simulink model "boris"  (R2020b)
settings: Solver=ode5  StartTime=0.0  StopTime=inf  FixedStep=1.0  RelTol=1e-3  EnableMultiTasking=on
libraries: simulink_extras x8
settings Model: Creator=Administrator  LastModifiedBy=boris
settings DataIOCC: LimitDataPoints=on  SaveFormat=Array  SignalLoggingSaveFormat=ModelDataLogs  ReturnWorkspaceOutputs=off
settings OptimizationCC: InitFltsAndDblsToZero=on  LifeSpan=inf
settings DebuggingCC: SaveWithParameterizedLinksMsg=none  UnderspecifiedInitializationDetection=Classic  MergeDetectMultiDrivingBlocksExec=none  SignalResolutionControl=TryResolveAllWithWarning  SolverPrmCheckMsg=warning  FcnCallInpInsideContextMsg=warning  SFUnexpectedBacktrackingDiag=warning  SFNoUnconditionalDefaultTransitionDiag=warning  SFExecutionAtInitializationDiag=none  ArithmeticOperatorsInVariantConditions=warning
settings HardwareCC: ProdBitPerPointer=32  ProdBitPerSizeT=32  ProdBitPerPtrDiffT=32  ProdLargestAtomicFloat=None  ProdIntDivRoundTo=Undefined  ProdEndianess=Unspecified  ProdWordSize=32  ProdHWDeviceType=32-bit Generic  TargetHWDeviceType=32-bit Generic
settings ModelReferenceCC: PropagateSignalLabelsOutOfModel=off
settings SFSimCC: SimUseLocalCustomCode=off  CustomCodeUndefinedFunction=UseInterfaceOnly
settings RTWCC: RTWUseLocalCustomCode=off
settings CodeAppCC: StateflowObjectComments=on
settings GRTTargetCC: TargetFcnLib=ansi_tfl_tmw.mat  TargetLangStandard=C89/C90 (ANSI)  CombineOutputUpdateFcns=off  GRTInterface=on
settings ConfigComp: CovMetricSettings=dw  CovSaveCumulativeToWorkspaceVar=on  CovSaveSingleToWorkspaceVar=on  CovExternalEMLEnable=off

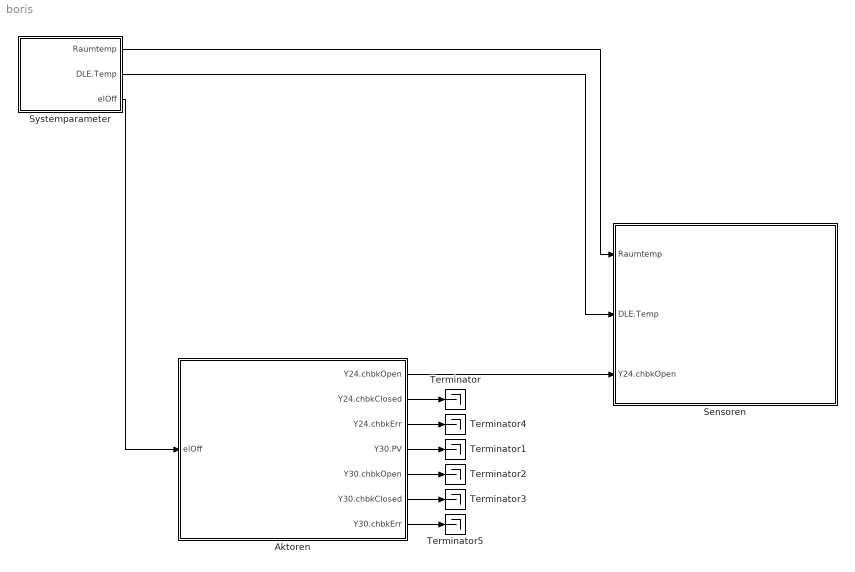
== system boris ==
  Aktoren : Subsystem  TreatAsAtomicUnit=on
  Sensoren : Subsystem  TreatAsAtomicUnit=on
  Systemparameter : Subsystem  TreatAsAtomicUnit=on
  Terminator{,1..5} (6 alike) : Terminator
  wires:
  Systemparameter/3(elOff) -> Aktoren/1(elOff)
  Systemparameter/2(DLE.Temp) -> Sensoren/2(DLE.Temp)
  Systemparameter/1(Raumtemp) -> Sensoren/1(Raumtemp)
  Aktoren/1(Y24.chbkOpen) -> Sensoren/3(Y24.chbkOpen)
  Aktoren/2(Y24.chbkClosed) -> Terminator/1
  Aktoren/4(Y30.PV) -> Terminator1/1
  Aktoren/5(Y30.chbkOpen) -> Terminator2/1
  Aktoren/6(Y30.chbkClosed) -> Terminator3/1
  Aktoren/3(Y24.chbkErr) -> Terminator4/1
  Aktoren/7(Y30.chbkErr) -> Terminator5/1

== system boris/Aktoren ==
  elOff : Inport  OutDataTypeStr=boolean
  Pumpen : Subsystem  TreatAsAtomicUnit=on
  Ventile : Subsystem  TreatAsAtomicUnit=on
  Y24.chbkOpen : Outport  OutDataTypeStr=boolean
  Y24.chbkClosed : Outport  Port=2  OutDataTypeStr=boolean
  Y24.chbkErr : Outport  Port=3  OutDataTypeStr=boolean
  Y30.PV : Outport  Port=4  OutDataTypeStr=double
  Y30.chbkOpen : Outport  Port=5  OutDataTypeStr=boolean
  Y30.chbkClosed : Outport  Port=6  OutDataTypeStr=boolean
  Y30.chbkErr : Outport  Port=7  OutDataTypeStr=boolean
  wires:
  elOff/1 -> Ventile/1(elOff), Pumpen/1(elOff)
  Ventile/1(Y24.chbkOpen) -> Y24.chbkOpen/1
  Ventile/2(Y24.chbkClosed) -> Y24.chbkClosed/1
  Ventile/4(Y30.PV) -> Y30.PV/1
  Ventile/6(Y30.chbkClosed) -> Y30.chbkClosed/1
  Ventile/5(Y30.chbkOpen) -> Y30.chbkOpen/1
  Ventile/3(Y24.chbkErr) -> Y24.chbkErr/1
  Ventile/7(Y30.chbkErr) -> Y30.chbkErr/1

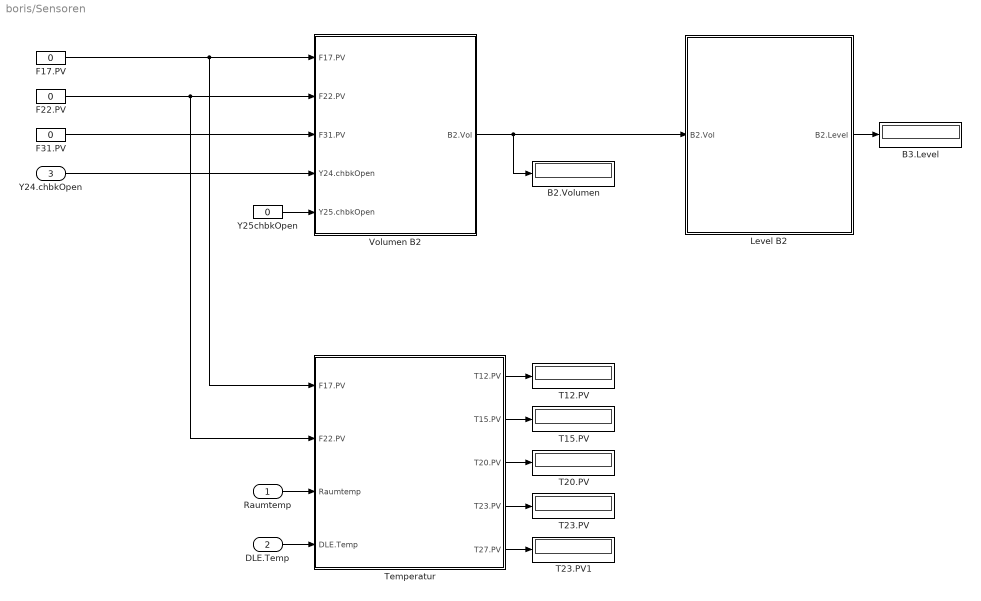
== system boris/Sensoren ==
  Raumtemp : Inport  OutDataTypeStr=double
  DLE.Temp : Inport  Port=2  OutDataTypeStr=double
  Y24.chbkOpen : Inport  Port=3  OutDataTypeStr=boolean
  B2.Volumen : Display
  B3.Level : Display
  F17.PV : Constant  Value=0  OutDataTypeStr=double
  F22.PV : Constant  Value=0  OutDataTypeStr=double
  F31.PV : Constant  Value=0  OutDataTypeStr=double
  Level B2 : Subsystem
  T12.PV : Display
  T15.PV : Display
  T20.PV : Display
  T23.PV : Display
  T23.PV1 : Display
  Temperatur : Subsystem
  Volumen B2 : Subsystem
  Y25chbkOpen : Constant  Value=0  OutDataTypeStr=boolean
  wires:
  Volumen B2/1(B2.Vol) -> Level B2/1(B2.Vol), B2.Volumen/1
  Raumtemp/1 -> Temperatur/3(Raumtemp)
  DLE.Temp/1 -> Temperatur/4(DLE.Temp)
  F17.PV/1 -> Volumen B2/1(F17.PV), Temperatur/1(F17.PV)
  F22.PV/1 -> Volumen B2/2(F22.PV), Temperatur/2(F22.PV)
  Y25chbkOpen/1 -> Volumen B2/5(Y25.chbkOpen)
  Temperatur/1(T12.PV) -> T12.PV/1
  Temperatur/2(T15.PV) -> T15.PV/1
  Temperatur/3(T20.PV) -> T20.PV/1
  Temperatur/4(T23.PV) -> T23.PV/1
  Level B2/1(B2.Level) -> B3.Level/1
  Y24.chbkOpen/1 -> Volumen B2/4(Y24.chbkOpen)
  F31.PV/1 -> Volumen B2/3(F31.PV)
  Temperatur/5(T27.PV) -> T23.PV1/1

== system boris/Systemparameter ==
  Ausfallwahrscheinlichkeit Stromversorgung : Constant  Value=0  OutDataTypeStr=double
  Ausgefallene Stromversorgung reparieren : Constant  Value=0  OutDataTypeStr=boolean
  Notaus : Constant  OutDataTypeStr=boolean
  Power : Constant  OutDataTypeStr=boolean
  Raumtemperatur : Constant  Value=20  OutDataTypeStr=double
  Strom aus? : Subsystem
  Temperatur Durchflauferhitzer : Constant  Value=40  OutDataTypeStr=double
  Raumtemp : Outport  OutDataTypeStr=double
  DLE.Temp : Outport  Port=2  OutDataTypeStr=double
  elOff : Outport  Port=3  OutDataTypeStr=boolean
  wires:
  Raumtemperatur/1 -> Raumtemp/1  "Raumtemp"
  Temperatur Durchflauferhitzer/1 -> DLE.Temp/1  "DLE.Temp"
  Notaus/1 -> Strom aus?/1(ilSSw)
  Power/1 -> Strom aus?/2(power)
  Ausfallwahrscheinlichkeit Stromversorgung/1 -> Strom aus?/3(pErrPow)
  Ausgefallene Stromversorgung reparieren/1 -> Strom aus?/4(PowRepai)
  Strom aus?/1(elOff) -> elOff/1  "elOff"

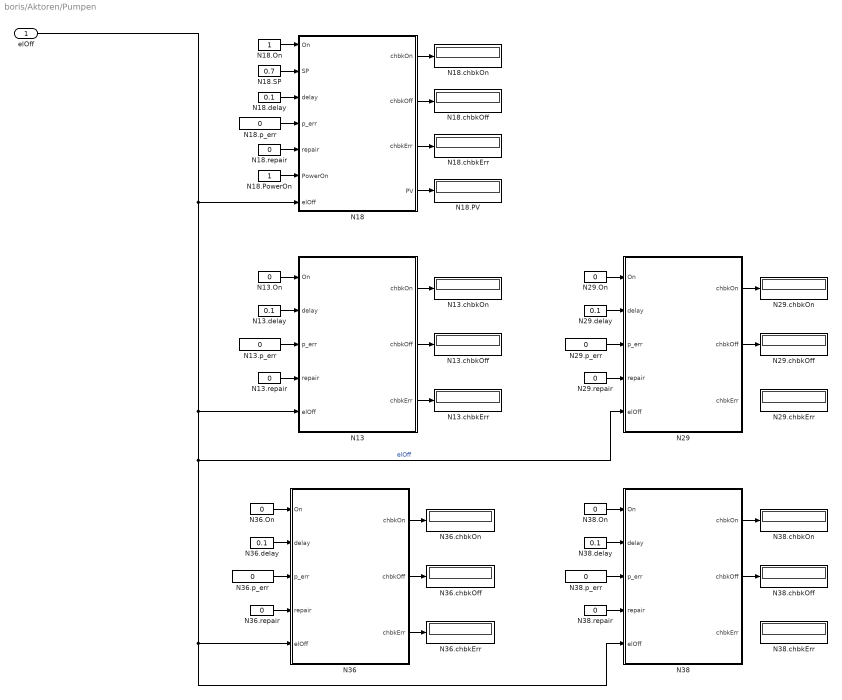
== system boris/Aktoren/Pumpen ==
  elOff : Inport  OutDataTypeStr=boolean
  N13 : Subsystem
  N13.On : Constant  Value=0  OutDataTypeStr=boolean
  N13.chbkErr : Display
  N13.chbkOff : Display
  N13.chbkOn : Display
  N13.delay : Constant  Value=0.1  OutDataTypeStr=double
  N13.p_err : Constant  Value=0  OutDataTypeStr=double
  N13.repair : Constant  Value=0  OutDataTypeStr=boolean
  N18 : Subsystem
  N18.On : Constant  OutDataTypeStr=boolean
  N18.PV : Display
  N18.PowerOn : Constant  OutDataTypeStr=boolean
  N18.SP : Constant  Value=0.7  OutDataTypeStr=double
  N18.chbkErr : Display
  N18.chbkOff : Display
  N18.chbkOn : Display
  N18.delay : Constant  Value=0.1  OutDataTypeStr=double
  N18.p_err : Constant  Value=0  OutDataTypeStr=double
  N18.repair : Constant  Value=0  OutDataTypeStr=boolean
  N29 : Subsystem
  N29.On : Constant  Value=0  OutDataTypeStr=boolean
  N29.chbkErr : Display
  N29.chbkOff : Display
  N29.chbkOn : Display
  N29.delay : Constant  Value=0.1  OutDataTypeStr=double
  N29.p_err : Constant  Value=0  OutDataTypeStr=double
  N29.repair : Constant  Value=0  OutDataTypeStr=boolean
  N36 : Subsystem
  N36.On : Constant  Value=0  OutDataTypeStr=boolean
  N36.chbkErr : Display
  N36.chbkOff : Display
  N36.chbkOn : Display
  N36.delay : Constant  Value=0.1  OutDataTypeStr=double
  N36.p_err : Constant  Value=0  OutDataTypeStr=double
  N36.repair : Constant  Value=0  OutDataTypeStr=boolean
  N38 : Subsystem
  N38.On : Constant  Value=0  OutDataTypeStr=boolean
  N38.chbkErr : Display
  N38.chbkOff : Display
  N38.chbkOn : Display
  N38.delay : Constant  Value=0.1  OutDataTypeStr=double
  N38.p_err : Constant  Value=0  OutDataTypeStr=double
  N38.repair : Constant  Value=0  OutDataTypeStr=boolean
  wires:
  N18/1(chbkOn) -> N18.chbkOn/1
  N18/2(chbkOff) -> N18.chbkOff/1
  N18/3(chbkErr) -> N18.chbkErr/1
  N18/4(PV) -> N18.PV/1
  N18.On/1 -> N18/1(On)
  N18.SP/1 -> N18/2(SP)
  N18.delay/1 -> N18/3(delay)
  N18.p_err/1 -> N18/4(p_err)
  N18.repair/1 -> N18/5(repair)
  N18.PowerOn/1 -> N18/6(PowerOn)
  N13/1(chbkOn) -> N13.chbkOn/1
  N13/2(chbkOff) -> N13.chbkOff/1
  N13.On/1 -> N13/1(On)
  N13.delay/1 -> N13/2(delay)
  N13.p_err/1 -> N13/3(p_err)
  N13.repair/1 -> N13/4(repair)
  N29/1(chbkOn) -> N29.chbkOn/1
  N29/2(chbkOff) -> N29.chbkOff/1
  ? -> N29.chbkErr/1
  N29.On/1 -> N29/1(On)
  N29.delay/1 -> N29/2(delay)
  N29.p_err/1 -> N29/3(p_err)
  N29.repair/1 -> N29/4(repair)
  N36/1(chbkOn) -> N36.chbkOn/1
  N36/2(chbkOff) -> N36.chbkOff/1
  N36/3(chbkErr) -> N36.chbkErr/1
  N36.On/1 -> N36/1(On)
  N36.delay/1 -> N36/2(delay)
  N36.p_err/1 -> N36/3(p_err)
  N36.repair/1 -> N36/4(repair)
  N38/1(chbkOn) -> N38.chbkOn/1
  N38/2(chbkOff) -> N38.chbkOff/1
  ? -> N38.chbkErr/1
  N38.On/1 -> N38/1(On)
  N38.delay/1 -> N38/2(delay)
  N38.p_err/1 -> N38/3(p_err)
  N38.repair/1 -> N38/4(repair)
  elOff/1 -> N13/5(elOff), N29/5(elOff), N36/5(elOff), N38/5(elOff), N18/7(elOff)  "elOff"
  N13/3(chbkErr) -> N13.chbkErr/1

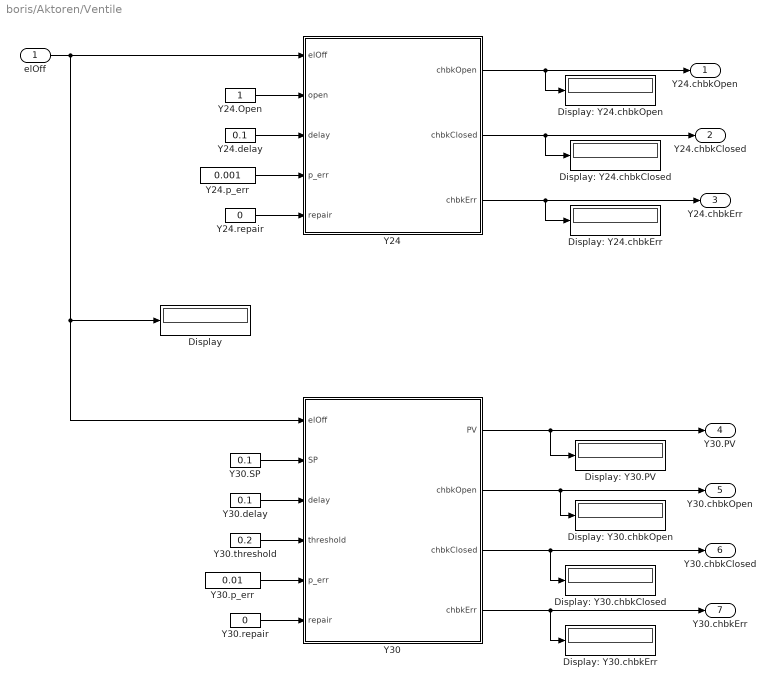
== system boris/Aktoren/Ventile ==
  elOff : Inport  OutDataTypeStr=boolean
  Display : Display
  Display: Y24.chbkClosed : Display
  Display: Y24.chbkErr : Display
  Display: Y24.chbkOpen : Display
  Display: Y30.PV : Display
  Display: Y30.chbkClosed : Display
  Display: Y30.chbkErr : Display
  Display: Y30.chbkOpen : Display
  Y24 : Subsystem
  Y24.Open : Constant  OutDataTypeStr=boolean
  Y24.delay : Constant  Value=0.1  OutDataTypeStr=double
  Y24.p_err : Constant  Value=0.001  OutDataTypeStr=double
  Y24.repair : Constant  Value=0  OutDataTypeStr=boolean
  Y30 : Subsystem
  Y30.SP : Constant  Value=0.1  OutDataTypeStr=double
  Y30.delay : Constant  Value=0.1  OutDataTypeStr=double
  Y30.p_err : Constant  Value=0.01  OutDataTypeStr=double
  Y30.repair : Constant  Value=0  OutDataTypeStr=boolean
  Y30.threshold : Constant  Value=0.2  OutDataTypeStr=double
  Y24.chbkOpen : Outport  OutDataTypeStr=boolean
  Y24.chbkClosed : Outport  Port=2  OutDataTypeStr=boolean
  Y24.chbkErr : Outport  Port=3  OutDataTypeStr=boolean
  Y30.PV : Outport  Port=4  OutDataTypeStr=double
  Y30.chbkOpen : Outport  Port=5  OutDataTypeStr=boolean
  Y30.chbkClosed : Outport  Port=6  OutDataTypeStr=boolean
  Y30.chbkErr : Outport  Port=7  OutDataTypeStr=boolean
  wires:
  elOff/1 -> Y24/1(elOff), Display/1, Y30/1(elOff)
  Y24.Open/1 -> Y24/2(open)
  Y24.delay/1 -> Y24/3(delay)
  Y24.p_err/1 -> Y24/4(p_err)
  Y24.repair/1 -> Y24/5(repair)
  Y30.SP/1 -> Y30/2(SP)
  Y30.delay/1 -> Y30/3(delay)
  Y30.p_err/1 -> Y30/5(p_err)
  Y30.repair/1 -> Y30/6(repair)
  Y30.threshold/1 -> Y30/4(threshold)
  Y24/1(chbkOpen) -> Display: Y24.chbkOpen/1, Y24.chbkOpen/1
  Y24/2(chbkClosed) -> Display: Y24.chbkClosed/1, Y24.chbkClosed/1
  Y30/1(PV) -> Display: Y30.PV/1, Y30.PV/1
  Y30/2(chbkOpen) -> Display: Y30.chbkOpen/1, Y30.chbkOpen/1
  Y30/3(chbkClosed) -> Display: Y30.chbkClosed/1, Y30.chbkClosed/1
  Y30/4(chbkErr) -> Display: Y30.chbkErr/1, Y30.chbkErr/1
  Y24/3(chbkErr) -> Display: Y24.chbkErr/1, Y24.chbkErr/1

== system boris/Sensoren/Level B2 ==
  B2.Vol : Inport
  B2.Level : Outport

== system boris/Sensoren/Temperatur ==
  F17.PV : Inport  OutDataTypeStr=double
  F22.PV : Inport  Port=2  OutDataTypeStr=double
  Raumtemp : Inport  Port=3  OutDataTypeStr=double
  DLE.Temp : Inport  Port=4  OutDataTypeStr=double
  T12.PV : Outport  OutDataTypeStr=double
  T15.PV : Outport  Port=2  OutDataTypeStr=double
  T20.PV : Outport  Port=3  OutDataTypeStr=double
  T23.PV : Outport  Port=4  OutDataTypeStr=double
  T27.PV : Outport  Port=5  OutDataTypeStr=double

== system boris/Sensoren/Volumen B2 ==
  F17.PV : Inport  OutDataTypeStr=double
  F22.PV : Inport  Port=2  OutDataTypeStr=double
  F31.PV : Inport  Port=3  OutDataTypeStr=double
  Y24.chbkOpen : Inport  Port=4  OutDataTypeStr=boolean
  Y25.chbkOpen : Inport  Port=5  OutDataTypeStr=boolean
  B2.Vol : Outport

== system boris/Systemparameter/Strom aus? ==
  ilSSw : Inport
  power : Inport  Port=2
  pErrPow : Inport  Port=3  OutDataTypeStr=double
  PowRepai : Inport  Port=4  OutDataTypeStr=boolean
  Logical Operator : Logic  AllPortsSameDT=off  OutDataTypeStr=boolean
  Logical Operator1 : Logic  Operator=NOT  AllPortsSameDT=off  OutDataTypeStr=boolean
  Notaus? : Subsystem  TreatAsAtomicUnit=on
  Stromausfall? : Subsystem  TreatAsAtomicUnit=on
  elOff : Outport  OutDataTypeStr=boolean
  wires:
  pErrPow/1 -> Stromausfall?/2(p_err)
  power/1 -> Stromausfall?/1(power), Notaus?/2(power)
  ilSSw/1 -> Notaus?/1(ilSSw)
  Logical Operator/1 -> Logical Operator1/1
  Notaus?/1(elOn) -> Logical Operator/1
  Stromausfall?/1(pow) -> Logical Operator/2
  PowRepai/1 -> Stromausfall?/3(repair)
  Logical Operator1/1 -> elOff/1

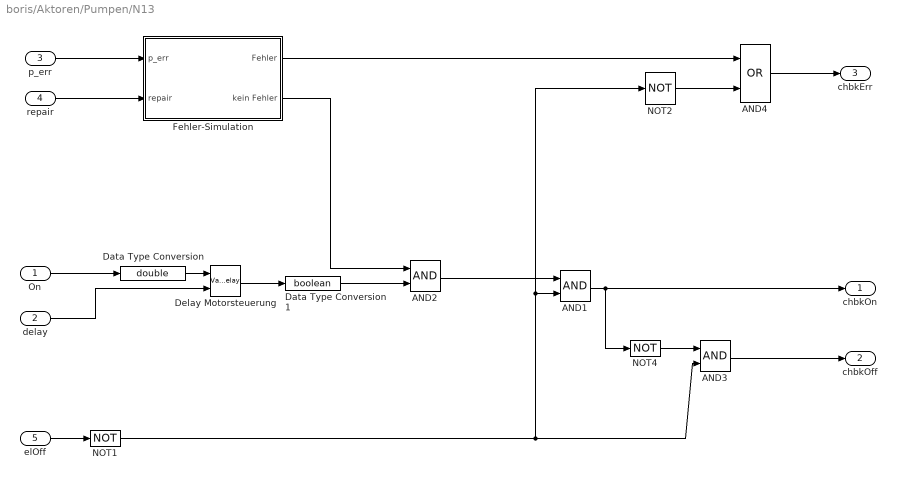
== system boris/Aktoren/Pumpen/N13 ==
  On : Inport  OutDataTypeStr=boolean
  delay : Inport  Port=2  OutDataTypeStr=double
  p_err : Inport  Port=3  OutDataTypeStr=double
  repair : Inport  Port=4  OutDataTypeStr=boolean
  elOff : Inport  Port=5  OutDataTypeStr=boolean
  AND1 : Logic  AllPortsSameDT=off  OutDataTypeStr=boolean
  AND2 : Logic  AllPortsSameDT=off  OutDataTypeStr=boolean
  AND3 : Logic  AllPortsSameDT=off  OutDataTypeStr=boolean
  AND4 : Logic  Operator=OR  AllPortsSameDT=off  OutDataTypeStr=boolean
  Data Type Conversion : DataTypeConversion  OutDataTypeStr=double
  Data Type Conversion1 : DataTypeConversion  OutDataTypeStr=boolean
  Delay Motorsteuerung : VariableTransportDelay  MaximumDelay=10  FixedBuffer=on
  Fehler-Simulation : Subsystem  TreatAsAtomicUnit=on
  NOT1 : Logic  Operator=NOT  AllPortsSameDT=off  OutDataTypeStr=boolean
  NOT2 : Logic  Operator=NOT  AllPortsSameDT=off  OutDataTypeStr=boolean
  NOT4 : Logic  Operator=NOT  AllPortsSameDT=off  OutDataTypeStr=boolean
  chbkOn : Outport  OutDataTypeStr=boolean
  chbkOff : Outport  Port=2  OutDataTypeStr=boolean
  chbkErr : Outport  Port=3  OutDataTypeStr=boolean
  wires:
  delay/1 -> Delay Motorsteuerung/2
  On/1 -> Data Type Conversion/1
  Delay Motorsteuerung/1 -> Data Type Conversion1/1
  Data Type Conversion/1 -> Delay Motorsteuerung/1
  Data Type Conversion1/1 -> AND2/2
  p_err/1 -> Fehler-Simulation/1(p_err)
  repair/1 -> Fehler-Simulation/2(repair)
  elOff/1 -> NOT1/1
  NOT1/1 -> AND3/2, AND1/2, NOT2/1
  AND2/1 -> AND1/1
  AND1/1 -> NOT4/1, chbkOn/1
  NOT4/1 -> AND3/1
  AND3/1 -> chbkOff/1
  Fehler-Simulation/2(kein Fehler) -> AND2/1
  AND4/1 -> chbkErr/1
  NOT2/1 -> AND4/2
  Fehler-Simulation/1(Fehler) -> AND4/1

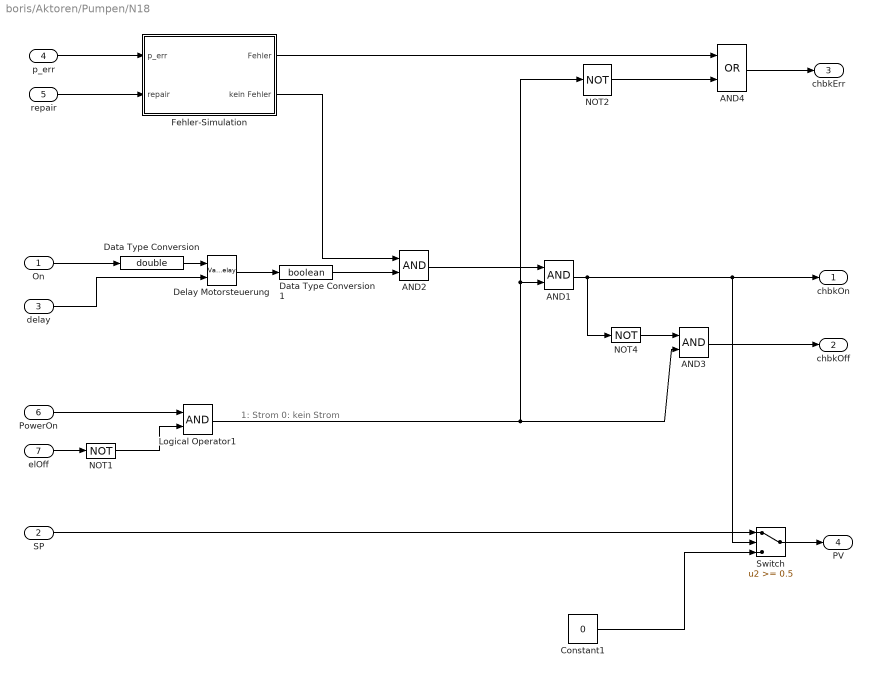
== system boris/Aktoren/Pumpen/N18 ==
  note: 1: Strom
      | 0: kein Strom
  On : Inport  OutDataTypeStr=boolean
  SP : Inport  Port=2  OutDataTypeStr=double
  delay : Inport  Port=3  OutDataTypeStr=double
  p_err : Inport  Port=4  OutDataTypeStr=double
  repair : Inport  Port=5  OutDataTypeStr=boolean
  PowerOn : Inport  Port=6  OutDataTypeStr=boolean
  elOff : Inport  Port=7  OutDataTypeStr=boolean
  AND1 : Logic  AllPortsSameDT=off  OutDataTypeStr=boolean
  AND2 : Logic  AllPortsSameDT=off  OutDataTypeStr=boolean
  AND3 : Logic  AllPortsSameDT=off  OutDataTypeStr=boolean
  AND4 : Logic  Operator=OR  AllPortsSameDT=off  OutDataTypeStr=boolean
  Constant1 : Constant  Value=0
  Data Type Conversion : DataTypeConversion  OutDataTypeStr=double
  Data Type Conversion1 : DataTypeConversion  OutDataTypeStr=boolean
  Delay Motorsteuerung : VariableTransportDelay  MaximumDelay=10  FixedBuffer=on
  Fehler-Simulation : Subsystem  TreatAsAtomicUnit=on
  Logical Operator1 : Logic  AllPortsSameDT=off  OutDataTypeStr=boolean
  NOT1 : Logic  Operator=NOT  AllPortsSameDT=off  OutDataTypeStr=boolean
  NOT2 : Logic  Operator=NOT  AllPortsSameDT=off  OutDataTypeStr=boolean
  NOT4 : Logic  Operator=NOT  AllPortsSameDT=off  OutDataTypeStr=boolean
  Switch : Switch  Threshold=0.5
  chbkOn : Outport  OutDataTypeStr=boolean
  chbkOff : Outport  Port=2  OutDataTypeStr=boolean
  chbkErr : Outport  Port=3  OutDataTypeStr=boolean
  PV : Outport  Port=4  OutDataTypeStr=double
  wires:
  delay/1 -> Delay Motorsteuerung/2
  On/1 -> Data Type Conversion/1
  Delay Motorsteuerung/1 -> Data Type Conversion1/1
  Logical Operator1/1 -> AND3/2, AND1/2, NOT2/1
  Data Type Conversion/1 -> Delay Motorsteuerung/1
  Data Type Conversion1/1 -> AND2/2
  p_err/1 -> Fehler-Simulation/1(p_err)
  repair/1 -> Fehler-Simulation/2(repair)
  PowerOn/1 -> Logical Operator1/1
  elOff/1 -> NOT1/1
  NOT1/1 -> Logical Operator1/2
  AND2/1 -> AND1/1
  AND1/1 -> NOT4/1, chbkOn/1, Switch/2
  NOT4/1 -> AND3/1
  AND3/1 -> chbkOff/1
  Fehler-Simulation/2(kein Fehler) -> AND2/1
  AND4/1 -> chbkErr/1
  Constant1/1 -> Switch/3
  Switch/1 -> PV/1
  SP/1 -> Switch/1
  NOT2/1 -> AND4/2
  Fehler-Simulation/1(Fehler) -> AND4/1

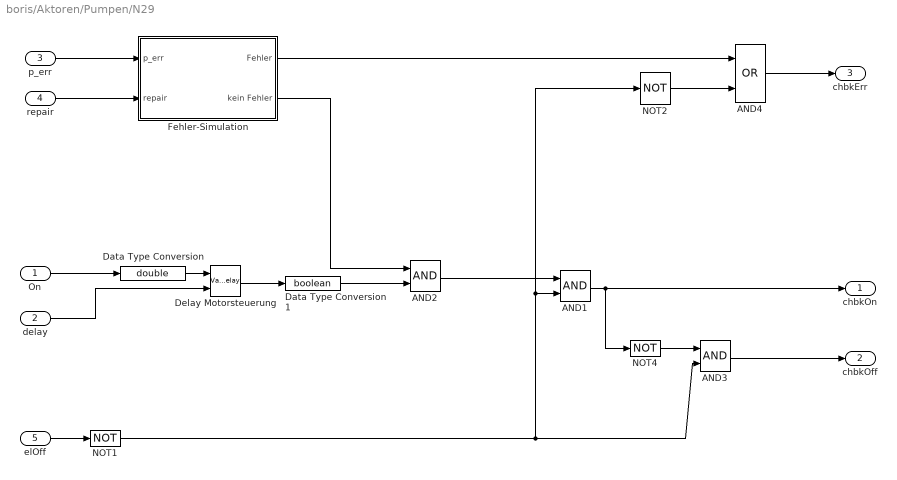
== system boris/Aktoren/Pumpen/N29 ==
  On : Inport  OutDataTypeStr=boolean
  delay : Inport  Port=2  OutDataTypeStr=double
  p_err : Inport  Port=3  OutDataTypeStr=double
  repair : Inport  Port=4  OutDataTypeStr=boolean
  elOff : Inport  Port=5  OutDataTypeStr=boolean
  AND1 : Logic  AllPortsSameDT=off  OutDataTypeStr=boolean
  AND2 : Logic  AllPortsSameDT=off  OutDataTypeStr=boolean
  AND3 : Logic  AllPortsSameDT=off  OutDataTypeStr=boolean
  AND4 : Logic  Operator=OR  AllPortsSameDT=off  OutDataTypeStr=boolean
  Data Type Conversion : DataTypeConversion  OutDataTypeStr=double
  Data Type Conversion1 : DataTypeConversion  OutDataTypeStr=boolean
  Delay Motorsteuerung : VariableTransportDelay  MaximumDelay=10  FixedBuffer=on
  Fehler-Simulation : Subsystem  TreatAsAtomicUnit=on
  NOT1 : Logic  Operator=NOT  AllPortsSameDT=off  OutDataTypeStr=boolean
  NOT2 : Logic  Operator=NOT  AllPortsSameDT=off  OutDataTypeStr=boolean
  NOT4 : Logic  Operator=NOT  AllPortsSameDT=off  OutDataTypeStr=boolean
  chbkOn : Outport  OutDataTypeStr=boolean
  chbkOff : Outport  Port=2  OutDataTypeStr=boolean
  chbkErr : Outport  Port=3  OutDataTypeStr=boolean
  wires:
  delay/1 -> Delay Motorsteuerung/2
  On/1 -> Data Type Conversion/1
  Delay Motorsteuerung/1 -> Data Type Conversion1/1
  Data Type Conversion/1 -> Delay Motorsteuerung/1
  Data Type Conversion1/1 -> AND2/2
  p_err/1 -> Fehler-Simulation/1(p_err)
  repair/1 -> Fehler-Simulation/2(repair)
  elOff/1 -> NOT1/1
  NOT1/1 -> AND3/2, AND1/2, NOT2/1
  AND2/1 -> AND1/1
  AND1/1 -> NOT4/1, chbkOn/1
  NOT4/1 -> AND3/1
  AND3/1 -> chbkOff/1
  Fehler-Simulation/2(kein Fehler) -> AND2/1
  AND4/1 -> chbkErr/1
  NOT2/1 -> AND4/2
  Fehler-Simulation/1(Fehler) -> AND4/1

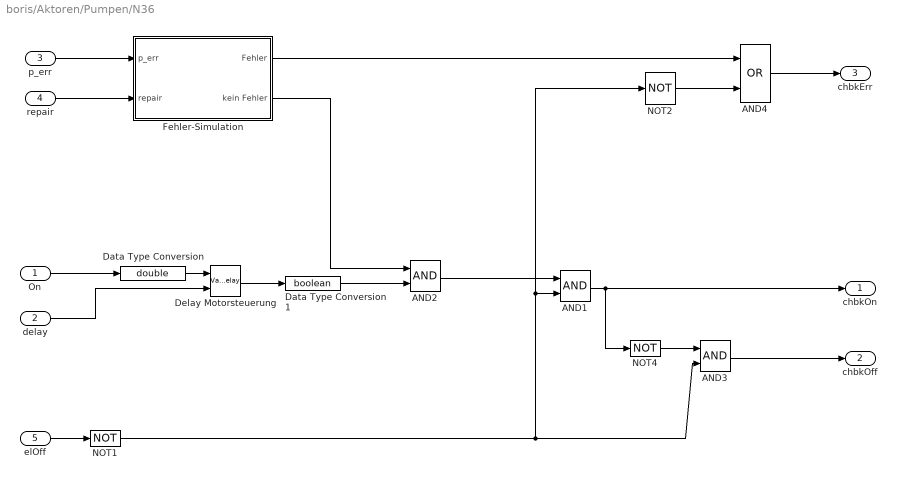
== system boris/Aktoren/Pumpen/N36 ==
  On : Inport  OutDataTypeStr=boolean
  delay : Inport  Port=2  OutDataTypeStr=double
  p_err : Inport  Port=3  OutDataTypeStr=double
  repair : Inport  Port=4  OutDataTypeStr=boolean
  elOff : Inport  Port=5  OutDataTypeStr=boolean
  AND1 : Logic  AllPortsSameDT=off  OutDataTypeStr=boolean
  AND2 : Logic  AllPortsSameDT=off  OutDataTypeStr=boolean
  AND3 : Logic  AllPortsSameDT=off  OutDataTypeStr=boolean
  AND4 : Logic  Operator=OR  AllPortsSameDT=off  OutDataTypeStr=boolean
  Data Type Conversion : DataTypeConversion  OutDataTypeStr=double
  Data Type Conversion1 : DataTypeConversion  OutDataTypeStr=boolean
  Delay Motorsteuerung : VariableTransportDelay  MaximumDelay=10  FixedBuffer=on
  Fehler-Simulation : Subsystem  TreatAsAtomicUnit=on
  NOT1 : Logic  Operator=NOT  AllPortsSameDT=off  OutDataTypeStr=boolean
  NOT2 : Logic  Operator=NOT  AllPortsSameDT=off  OutDataTypeStr=boolean
  NOT4 : Logic  Operator=NOT  AllPortsSameDT=off  OutDataTypeStr=boolean
  chbkOn : Outport  OutDataTypeStr=boolean
  chbkOff : Outport  Port=2  OutDataTypeStr=boolean
  chbkErr : Outport  Port=3  OutDataTypeStr=boolean
  wires:
  delay/1 -> Delay Motorsteuerung/2
  On/1 -> Data Type Conversion/1
  Delay Motorsteuerung/1 -> Data Type Conversion1/1
  Data Type Conversion/1 -> Delay Motorsteuerung/1
  Data Type Conversion1/1 -> AND2/2
  p_err/1 -> Fehler-Simulation/1(p_err)
  repair/1 -> Fehler-Simulation/2(repair)
  elOff/1 -> NOT1/1
  NOT1/1 -> AND3/2, AND1/2, NOT2/1
  AND2/1 -> AND1/1
  AND1/1 -> NOT4/1, chbkOn/1
  NOT4/1 -> AND3/1
  AND3/1 -> chbkOff/1
  Fehler-Simulation/2(kein Fehler) -> AND2/1
  AND4/1 -> chbkErr/1
  NOT2/1 -> AND4/2
  Fehler-Simulation/1(Fehler) -> AND4/1

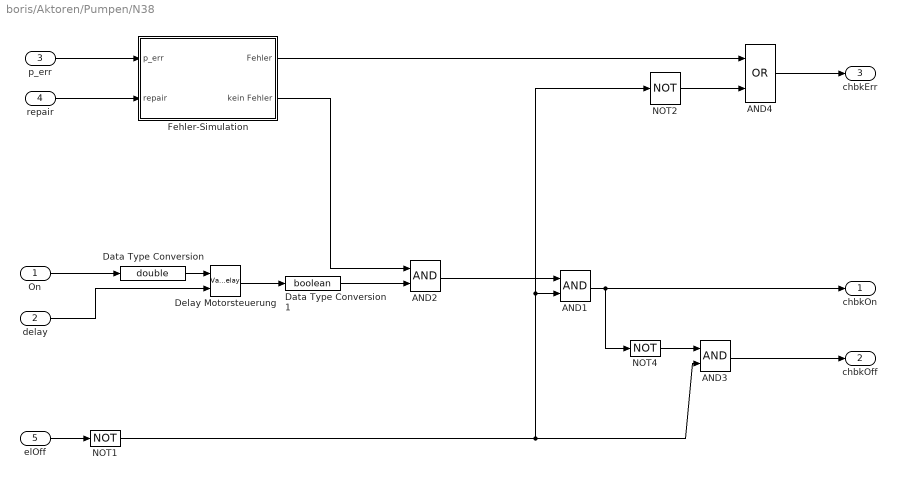
== system boris/Aktoren/Pumpen/N38 ==
  On : Inport  OutDataTypeStr=boolean
  delay : Inport  Port=2  OutDataTypeStr=double
  p_err : Inport  Port=3  OutDataTypeStr=double
  repair : Inport  Port=4  OutDataTypeStr=boolean
  elOff : Inport  Port=5  OutDataTypeStr=boolean
  AND1 : Logic  AllPortsSameDT=off  OutDataTypeStr=boolean
  AND2 : Logic  AllPortsSameDT=off  OutDataTypeStr=boolean
  AND3 : Logic  AllPortsSameDT=off  OutDataTypeStr=boolean
  AND4 : Logic  Operator=OR  AllPortsSameDT=off  OutDataTypeStr=boolean
  Data Type Conversion : DataTypeConversion  OutDataTypeStr=double
  Data Type Conversion1 : DataTypeConversion  OutDataTypeStr=boolean
  Delay Motorsteuerung : VariableTransportDelay  MaximumDelay=10  FixedBuffer=on
  Fehler-Simulation : Subsystem  TreatAsAtomicUnit=on
  NOT1 : Logic  Operator=NOT  AllPortsSameDT=off  OutDataTypeStr=boolean
  NOT2 : Logic  Operator=NOT  AllPortsSameDT=off  OutDataTypeStr=boolean
  NOT4 : Logic  Operator=NOT  AllPortsSameDT=off  OutDataTypeStr=boolean
  chbkOn : Outport  OutDataTypeStr=boolean
  chbkOff : Outport  Port=2  OutDataTypeStr=boolean
  chbkErr : Outport  Port=3  OutDataTypeStr=boolean
  wires:
  delay/1 -> Delay Motorsteuerung/2
  On/1 -> Data Type Conversion/1
  Delay Motorsteuerung/1 -> Data Type Conversion1/1
  Data Type Conversion/1 -> Delay Motorsteuerung/1
  Data Type Conversion1/1 -> AND2/2
  p_err/1 -> Fehler-Simulation/1(p_err)
  repair/1 -> Fehler-Simulation/2(repair)
  elOff/1 -> NOT1/1
  NOT1/1 -> AND3/2, AND1/2, NOT2/1
  AND2/1 -> AND1/1
  AND1/1 -> NOT4/1, chbkOn/1
  NOT4/1 -> AND3/1
  AND3/1 -> chbkOff/1
  Fehler-Simulation/2(kein Fehler) -> AND2/1
  AND4/1 -> chbkErr/1
  NOT2/1 -> AND4/2
  Fehler-Simulation/1(Fehler) -> AND4/1

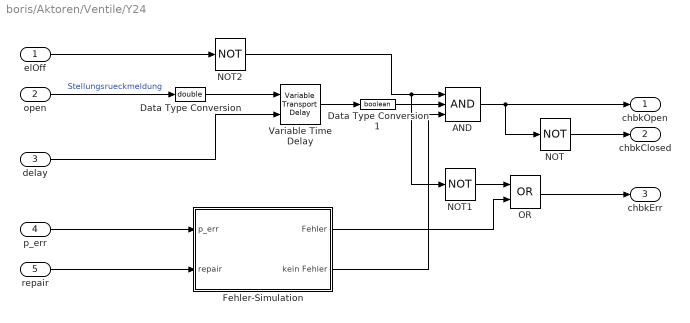
== system boris/Aktoren/Ventile/Y24 ==
  elOff : Inport  OutDataTypeStr=boolean
  open : Inport  Port=2  OutDataTypeStr=boolean
  delay : Inport  Port=3  OutDataTypeStr=double
  p_err : Inport  Port=4  OutDataTypeStr=double
  repair : Inport  Port=5  OutDataTypeStr=boolean
  AND : Logic  Inputs=3  AllPortsSameDT=off  OutDataTypeStr=boolean
  Data Type Conversion : DataTypeConversion  OutDataTypeStr=double
  Data Type Conversion1 : DataTypeConversion  OutDataTypeStr=boolean
  Fehler-Simulation : Subsystem  TreatAsAtomicUnit=on
  NOT : Logic  Operator=NOT  AllPortsSameDT=off  OutDataTypeStr=boolean
  NOT1 : Logic  Operator=NOT  AllPortsSameDT=off  OutDataTypeStr=boolean
  NOT2 : Logic  Operator=NOT  AllPortsSameDT=off  OutDataTypeStr=boolean
  OR : Logic  Operator=OR  AllPortsSameDT=off  OutDataTypeStr=boolean
  Variable Time Delay : VariableTransportDelay  VariableDelayType=Variable transport delay  MaximumDelay=10
  chbkOpen : Outport  OutDataTypeStr=boolean
  chbkClosed : Outport  Port=2  OutDataTypeStr=boolean
  chbkErr : Outport  Port=3  OutDataTypeStr=boolean
  wires:
  NOT/1 -> chbkClosed/1
  AND/1 -> chbkOpen/1, NOT/1
  delay/1 -> Variable Time Delay/2
  elOff/1 -> NOT2/1
  p_err/1 -> Fehler-Simulation/1(p_err)
  repair/1 -> Fehler-Simulation/2(repair)
  Data Type Conversion/1 -> Variable Time Delay/1
  Variable Time Delay/1 -> Data Type Conversion1/1
  Data Type Conversion1/1 -> AND/2
  open/1 -> Data Type Conversion/1  "Stellungsrueckmeldung"
  NOT1/1 -> OR/1
  Fehler-Simulation/1(Fehler) -> OR/2
  OR/1 -> chbkErr/1
  Fehler-Simulation/2(kein Fehler) -> AND/3
  NOT2/1 -> NOT1/1, AND/1

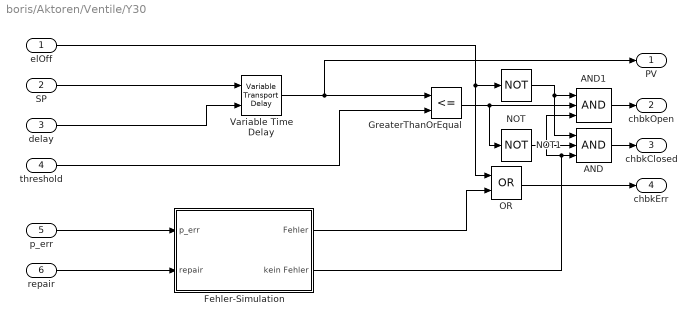
== system boris/Aktoren/Ventile/Y30 ==
  elOff : Inport  OutDataTypeStr=boolean
  SP : Inport  Port=2  OutDataTypeStr=double
  delay : Inport  Port=3  OutDataTypeStr=double
  threshold : Inport  Port=4  OutDataTypeStr=double
  p_err : Inport  Port=5  OutDataTypeStr=double
  repair : Inport  Port=6  OutDataTypeStr=boolean
  AND : Logic  Inputs=3  AllPortsSameDT=off  OutDataTypeStr=boolean
  AND1 : Logic  Inputs=3  AllPortsSameDT=off  OutDataTypeStr=boolean
  Fehler-Simulation : Subsystem  TreatAsAtomicUnit=on
  GreaterThanOrEqual : RelationalOperator  Operator=<=  OutDataTypeStr=boolean  RndMeth=Simplest
  NOT : Logic  Operator=NOT  AllPortsSameDT=off  OutDataTypeStr=boolean
  NOT1 : Logic  Operator=NOT  AllPortsSameDT=off  OutDataTypeStr=boolean
  OR : Logic  Operator=OR  AllPortsSameDT=off  OutDataTypeStr=boolean
  Variable Time Delay : VariableTransportDelay  MaximumDelay=10
  PV : Outport  OutDataTypeStr=double
  chbkOpen : Outport  Port=2  OutDataTypeStr=boolean
  chbkClosed : Outport  Port=3  OutDataTypeStr=boolean
  chbkErr : Outport  Port=4  OutDataTypeStr=boolean
  wires:
  p_err/1 -> Fehler-Simulation/1(p_err)
  repair/1 -> Fehler-Simulation/2(repair)
  Fehler-Simulation/2(kein Fehler) -> AND/3, AND1/3
  delay/1 -> Variable Time Delay/2
  Variable Time Delay/1 -> PV/1, GreaterThanOrEqual/1
  SP/1 -> Variable Time Delay/1
  OR/1 -> chbkErr/1
  Fehler-Simulation/1(Fehler) -> OR/2
  GreaterThanOrEqual/1 -> AND1/2, NOT1/1
  threshold/1 -> GreaterThanOrEqual/2
  AND/1 -> chbkClosed/1
  NOT1/1 -> AND/2
  AND1/1 -> chbkOpen/1
  elOff/1 -> NOT/1, OR/1
  NOT/1 -> AND/1, AND1/1

== system boris/Systemparameter/Strom aus?/Notaus? ==
  ilSSw : Inport
  power : Inport  Port=2
  Logical Operator : Logic  AllPortsSameDT=off  OutDataTypeStr=boolean
  elOn : Outport
  wires:
  Logical Operator/1 -> elOn/1
  ilSSw/1 -> Logical Operator/1
  power/1 -> Logical Operator/2

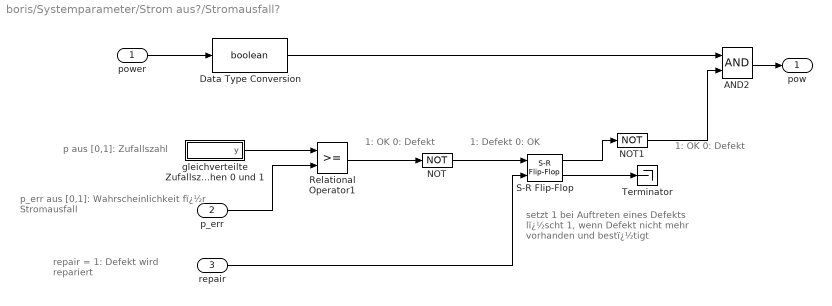
== system boris/Systemparameter/Strom aus?/Stromausfall? ==
  note: p_err aus [0,1]:
      | Wahrscheinlichkeit fï¿½r Stromausfall
  note: p aus [0,1]: Zufallszahl
  note: 1: OK
      | 0: Defekt
  note: 1: Defekt
      | 0: OK
  note: repair = 1:
      | Defekt wird repariert
  note: setzt 1 bei Auftreten eines Defekts
      | lï¿½scht 1, wenn Defekt nicht mehr
      |               vorhanden und bestï¿½tigt
  note: 1: OK
      | 0: Defekt
  power : Inport
  p_err : Inport  Port=2
  repair : Inport  Port=3  OutDataTypeStr=boolean
  AND2 : Logic  AllPortsSameDT=off  OutDataTypeStr=boolean
  Data Type Conversion : DataTypeConversion  OutDataTypeStr=boolean
  NOT : Logic  Operator=NOT  AllPortsSameDT=off  OutDataTypeStr=boolean
  NOT1 : Logic  Operator=NOT  AllPortsSameDT=off  OutDataTypeStr=boolean
  Relational Operator1 : RelationalOperator  OutDataTypeStr=boolean  RndMeth=Nearest
  S-R Flip-Flop : simulink_extras/Flip Flops/S-R Flip-Flop  initial_condition=0
  Terminator : Terminator
  gleichverteilte Zufallszahl zwischen 0 und 1 : MATLAB Function  TreatAsAtomicUnit=on
  pow : Outport
  wires:
  power/1 -> Data Type Conversion/1
  gleichverteilte Zufallszahl zwischen 0 und 1/1(y) -> Relational Operator1/1
  p_err/1 -> Relational Operator1/2
  AND2/1 -> pow/1
  Data Type Conversion/1 -> AND2/1
  repair/1 -> S-R Flip-Flop/2
  Relational Operator1/1 -> NOT/1
  NOT/1 -> S-R Flip-Flop/1
  S-R Flip-Flop/2 -> Terminator/1
  S-R Flip-Flop/1 -> NOT1/1
  NOT1/1 -> AND2/2

== system boris/Aktoren/Pumpen/N13/Fehler-Simulation ==
  note: 1: OK
      | 0: Defekt
  note: 1: Defekt
      | 0: OK
  p_err : Inport  OutDataTypeStr=double
  repair : Inport  Port=2  OutDataTypeStr=boolean
  Logical Operator : Logic  Operator=NOT  AllPortsSameDT=off  OutDataTypeStr=boolean
  NOT : Logic  Operator=NOT  AllPortsSameDT=off  OutDataTypeStr=boolean
  Relational Operator : RelationalOperator  OutDataTypeStr=boolean  RndMeth=Nearest
  S-R Flip-Flop : simulink_extras/Flip Flops/S-R Flip-Flop  initial_condition=0
  Terminator : Terminator
  Uniform Random Number : UniformRandomNumber  Minimum=0  Seed=1  SampleTime=1
  Fehler : Outport  OutDataTypeStr=boolean
  kein Fehler : Outport  Port=2  OutDataTypeStr=boolean
  wires:
  repair/1 -> S-R Flip-Flop/2
  Relational Operator/1 -> NOT/1
  Uniform Random Number/1 -> Relational Operator/1
  p_err/1 -> Relational Operator/2
  NOT/1 -> S-R Flip-Flop/1
  S-R Flip-Flop/1 -> Logical Operator/1, Fehler/1
  Logical Operator/1 -> kein Fehler/1
  S-R Flip-Flop/2 -> Terminator/1

== system boris/Aktoren/Pumpen/N18/Fehler-Simulation ==
  note: 1: OK
      | 0: Defekt
  note: 1: Defekt
      | 0: OK
  p_err : Inport  OutDataTypeStr=double
  repair : Inport  Port=2  OutDataTypeStr=boolean
  Logical Operator : Logic  Operator=NOT  AllPortsSameDT=off  OutDataTypeStr=boolean
  NOT : Logic  Operator=NOT  AllPortsSameDT=off  OutDataTypeStr=boolean
  Relational Operator : RelationalOperator  OutDataTypeStr=boolean  RndMeth=Nearest
  S-R Flip-Flop : simulink_extras/Flip Flops/S-R Flip-Flop  initial_condition=0
  Terminator : Terminator
  Uniform Random Number : UniformRandomNumber  Minimum=0  Seed=1  SampleTime=1
  Fehler : Outport  OutDataTypeStr=boolean
  kein Fehler : Outport  Port=2  OutDataTypeStr=boolean
  wires:
  repair/1 -> S-R Flip-Flop/2
  Relational Operator/1 -> NOT/1
  Uniform Random Number/1 -> Relational Operator/1
  p_err/1 -> Relational Operator/2
  NOT/1 -> S-R Flip-Flop/1
  S-R Flip-Flop/1 -> Logical Operator/1, Fehler/1
  Logical Operator/1 -> kein Fehler/1
  S-R Flip-Flop/2 -> Terminator/1

== system boris/Aktoren/Pumpen/N29/Fehler-Simulation ==
  note: 1: OK
      | 0: Defekt
  note: 1: Defekt
      | 0: OK
  p_err : Inport  OutDataTypeStr=double
  repair : Inport  Port=2  OutDataTypeStr=boolean
  Logical Operator : Logic  Operator=NOT  AllPortsSameDT=off  OutDataTypeStr=boolean
  NOT : Logic  Operator=NOT  AllPortsSameDT=off  OutDataTypeStr=boolean
  Relational Operator : RelationalOperator  OutDataTypeStr=boolean  RndMeth=Nearest
  S-R Flip-Flop : simulink_extras/Flip Flops/S-R Flip-Flop  initial_condition=0
  Terminator : Terminator
  Uniform Random Number : UniformRandomNumber  Minimum=0  Seed=1  SampleTime=1
  Fehler : Outport  OutDataTypeStr=boolean
  kein Fehler : Outport  Port=2  OutDataTypeStr=boolean
  wires:
  repair/1 -> S-R Flip-Flop/2
  Relational Operator/1 -> NOT/1
  Uniform Random Number/1 -> Relational Operator/1
  p_err/1 -> Relational Operator/2
  NOT/1 -> S-R Flip-Flop/1
  S-R Flip-Flop/1 -> Logical Operator/1, Fehler/1
  Logical Operator/1 -> kein Fehler/1
  S-R Flip-Flop/2 -> Terminator/1

== system boris/Aktoren/Pumpen/N36/Fehler-Simulation ==
  note: 1: OK
      | 0: Defekt
  note: 1: Defekt
      | 0: OK
  p_err : Inport  OutDataTypeStr=double
  repair : Inport  Port=2  OutDataTypeStr=boolean
  Logical Operator : Logic  Operator=NOT  AllPortsSameDT=off  OutDataTypeStr=boolean
  NOT : Logic  Operator=NOT  AllPortsSameDT=off  OutDataTypeStr=boolean
  Relational Operator : RelationalOperator  OutDataTypeStr=boolean  RndMeth=Nearest
  S-R Flip-Flop : simulink_extras/Flip Flops/S-R Flip-Flop  initial_condition=0
  Uniform Random Number : UniformRandomNumber  Minimum=0  Seed=1  SampleTime=1
  Fehler : Outport  OutDataTypeStr=boolean
  kein Fehler : Outport  Port=2  OutDataTypeStr=boolean
  wires:
  repair/1 -> S-R Flip-Flop/2
  Relational Operator/1 -> NOT/1
  Uniform Random Number/1 -> Relational Operator/1
  p_err/1 -> Relational Operator/2
  NOT/1 -> S-R Flip-Flop/1
  S-R Flip-Flop/1 -> Logical Operator/1, Fehler/1
  Logical Operator/1 -> kein Fehler/1

== system boris/Aktoren/Pumpen/N38/Fehler-Simulation ==
  note: 1: OK
      | 0: Defekt
  note: 1: Defekt
      | 0: OK
  p_err : Inport  OutDataTypeStr=double
  repair : Inport  Port=2  OutDataTypeStr=boolean
  Logical Operator : Logic  Operator=NOT  AllPortsSameDT=off  OutDataTypeStr=boolean
  NOT : Logic  Operator=NOT  AllPortsSameDT=off  OutDataTypeStr=boolean
  Relational Operator : RelationalOperator  OutDataTypeStr=boolean  RndMeth=Nearest
  S-R Flip-Flop : simulink_extras/Flip Flops/S-R Flip-Flop  initial_condition=0
  Uniform Random Number : UniformRandomNumber  Minimum=0  Seed=1  SampleTime=1
  Fehler : Outport  OutDataTypeStr=boolean
  kein Fehler : Outport  Port=2  OutDataTypeStr=boolean
  wires:
  repair/1 -> S-R Flip-Flop/2
  Relational Operator/1 -> NOT/1
  Uniform Random Number/1 -> Relational Operator/1
  p_err/1 -> Relational Operator/2
  NOT/1 -> S-R Flip-Flop/1
  S-R Flip-Flop/1 -> Logical Operator/1, Fehler/1
  Logical Operator/1 -> kein Fehler/1

== system boris/Aktoren/Ventile/Y24/Fehler-Simulation ==
  note: 1: OK
      | 0: Defekt
  note: 1: Defekt
      | 0: OK
  p_err : Inport  OutDataTypeStr=double
  repair : Inport  Port=2  OutDataTypeStr=boolean
  Logical Operator : Logic  Operator=NOT  AllPortsSameDT=off  OutDataTypeStr=boolean
  NOT : Logic  Operator=NOT  AllPortsSameDT=off  OutDataTypeStr=boolean
  Relational Operator : RelationalOperator  OutDataTypeStr=boolean  RndMeth=Nearest
  S-R Flip-Flop : simulink_extras/Flip Flops/S-R Flip-Flop  initial_condition=0
  Terminator : Terminator
  Uniform Random Number : UniformRandomNumber  Minimum=0  Seed=1  SampleTime=1
  Fehler : Outport  OutDataTypeStr=boolean
  kein Fehler : Outport  Port=2  OutDataTypeStr=boolean
  wires:
  repair/1 -> S-R Flip-Flop/2
  Relational Operator/1 -> NOT/1
  Uniform Random Number/1 -> Relational Operator/1
  p_err/1 -> Relational Operator/2
  NOT/1 -> S-R Flip-Flop/1
  S-R Flip-Flop/1 -> Logical Operator/1, Fehler/1
  Logical Operator/1 -> kein Fehler/1
  S-R Flip-Flop/2 -> Terminator/1

== system boris/Aktoren/Ventile/Y30/Fehler-Simulation ==
  note: 1: OK
      | 0: Defekt
  note: 1: Defekt
      | 0: OK
  p_err : Inport  OutDataTypeStr=double
  repair : Inport  Port=2  OutDataTypeStr=boolean
  Logical Operator : Logic  Operator=NOT  AllPortsSameDT=off  OutDataTypeStr=boolean
  NOT : Logic  Operator=NOT  AllPortsSameDT=off  OutDataTypeStr=boolean
  Relational Operator : RelationalOperator  OutDataTypeStr=boolean  RndMeth=Nearest
  S-R Flip-Flop : simulink_extras/Flip Flops/S-R Flip-Flop  initial_condition=0
  Terminator : Terminator
  Uniform Random Number : UniformRandomNumber  Minimum=0  Seed=1  SampleTime=1
  Fehler : Outport  OutDataTypeStr=boolean
  kein Fehler : Outport  Port=2  OutDataTypeStr=boolean
  wires:
  repair/1 -> S-R Flip-Flop/2
  Relational Operator/1 -> NOT/1
  Uniform Random Number/1 -> Relational Operator/1
  p_err/1 -> Relational Operator/2
  NOT/1 -> S-R Flip-Flop/1
  S-R Flip-Flop/1 -> Logical Operator/1, Fehler/1
  Logical Operator/1 -> kein Fehler/1
  S-R Flip-Flop/2 -> Terminator/1

== matlab function boris/Systemparameter/Strom aus?/Stromausfall?/gleichverteilte Zufallszahl zwischen 0 und 1 ==
  data: y output
function y = Zufall
% This block supports an embeddable subset of the MATLAB language.
% See the help menu for details. 

y = rand(1,1);
